simulink model "CTS_Control_Disturbance_Simulink"  (R2023a)
settings: Solver=VariableStepAuto  StartTime=0.0  StopTime=10.0  RelTol=1e-3
undefined symbols (not defined in the file): A_1, A_2, c_1, c_2, h_10, h_20, ICs, K, q_i0
settings Model: Creator=m260477  LastModifiedBy=m260477

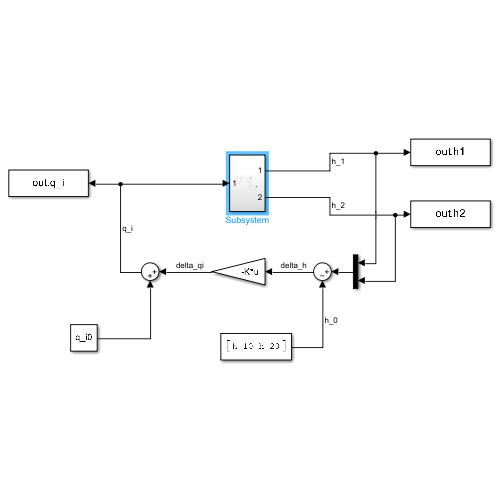
[thumbnail: Simulink's stored preview of the top-level diagram]
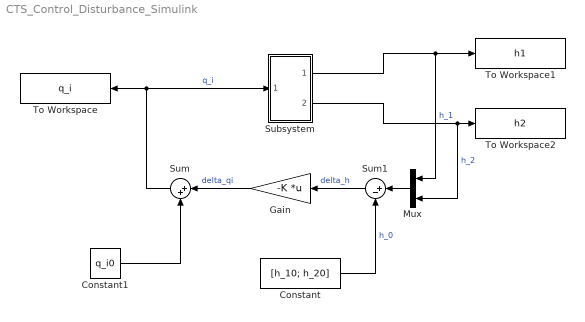
== system CTS_Control_Disturbance_Simulink ==
  Constant : Constant  Value=[h_10; h_20]
  Constant1 : Constant  Value=q_i0
  Gain : Gain  Gain=-K  Multiplication=Matrix(K*u)
  Mux : Mux  Inputs=2
  Subsystem : Subsystem
  Sum : Sum  Inputs=|++
  Sum1 : Sum  Inputs=|+-
  To Workspace : ToWorkspace  VariableName=q_i  SaveFormat=Timeseries  SampleTime=-1
  To Workspace1 : ToWorkspace  VariableName=h1  SaveFormat=Timeseries  SampleTime=-1
  To Workspace2 : ToWorkspace  VariableName=h2  SaveFormat=Timeseries  SampleTime=-1
  wires:
  Subsystem/1(Out1) -> Mux/1, To Workspace1/1  "h_1"
  Subsystem/2(Out3) -> Mux/2, To Workspace2/1  "h_2"
  Constant1/1 -> Sum/2
  Gain/1 -> Sum/1  "delta_qi"
  Sum1/1 -> Gain/1  "delta_h"
  Constant/1 -> Sum1/2  "h_0"
  Sum/1 -> Subsystem/1(Input), To Workspace/1  "q_i"
  Mux/1 -> Sum1/1

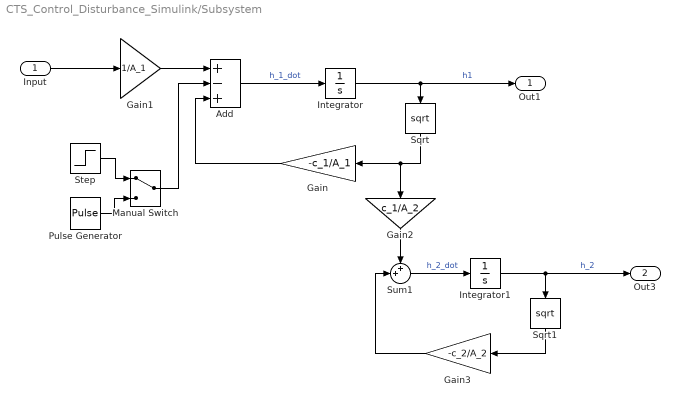
== system CTS_Control_Disturbance_Simulink/Subsystem ==
  Input : Inport
  Add : Sum  Inputs=+-+
  Gain : Gain  Gain=-c_1/A_1
  Gain1 : Gain  Gain=1/A_1
  Gain2 : Gain  Gain=c_1/A_2
  Gain3 : Gain  Gain=-c_2/A_2
  Integrator : Integrator  InitialCondition=ICs
  Integrator1 : Integrator  InitialCondition=ICs
  Manual Switch : ManualSwitch
  Pulse Generator : DiscretePulseGenerator  PulseType=Time based  Amplitude=0.3*q_i0  Period=100  PulseWidth=40  PhaseDelay=100
  Sqrt : Sqrt
  Sqrt1 : Sqrt
  Step : Step  Time=100  After=0.3*q_i0  SampleTime=0
  Sum1 : Sum  Inputs=++|
  Out1 : Outport
  Out3 : Outport  Port=2
  wires:
  Integrator1/1 -> Out3/1, Sqrt1/1  "h_2"
  Input/1 -> Gain1/1
  Gain1/1 -> Add/1
  Sqrt1/1 -> Gain3/1
  Gain2/1 -> Sum1/1
  Integrator/1 -> Out1/1, Sqrt/1  "h1"
  Add/1 -> Integrator/1  "h_1_dot"
  Gain3/1 -> Sum1/2
  Sum1/1 -> Integrator1/1  "h_2_dot"
  Gain/1 -> Add/3
  Sqrt/1 -> Gain2/1, Gain/1
  Step/1 -> Manual Switch/1
  Pulse Generator/1 -> Manual Switch/2
  Manual Switch/1 -> Add/2
